simulink model "regulering_model"  (R2019b)
settings: Solver=VariableStepAuto  StartTime=0.0  StopTime=10000  FixedStep=0.01  RelTol=1e-3
settings Model: Creator=oskar  LastModifiedBy=oskar

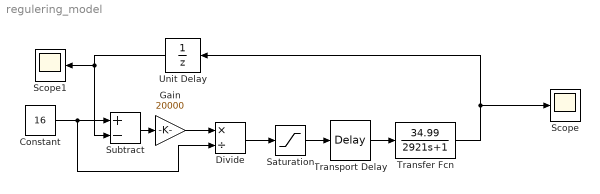
== system regulering_model ==
  Constant : Constant  Value=16
  Divide : Product  Inputs=*/
  Gain : Gain  Gain=20000
  Saturation : Saturate  UpperLimit=1  LowerLimit=0
  Scope : Scope
  Scope1 : Scope
  Subtract : Sum  Inputs=+-
  Transfer Fcn : TransferFcn  Numerator=[34.99]  Denominator=[2921 1]
  Transport Delay : TransportDelay
  Unit Delay : UnitDelay  SampleTime=0.1  HasFrameUpgradeWarning=on
  wires:
  Transfer Fcn/1 -> Unit Delay/1, Scope/1
  Constant/1 -> Divide/2, Subtract/1
  Subtract/1 -> Gain/1
  Saturation/1 -> Transport Delay/1
  Divide/1 -> Saturation/1
  Gain/1 -> Divide/1
  Unit Delay/1 -> Subtract/2, Scope1/1
  Transport Delay/1 -> Transfer Fcn/1
